simulink model "TransmissionController"  (R2026b)
StartFcn:
  | %tic
StopFcn:
  | %toc
libraries: autolibtranscontrolscommon x1
settings Model: Creator=The MathWorks, Inc.  LastModifiedBy=The MathWorks, Inc.

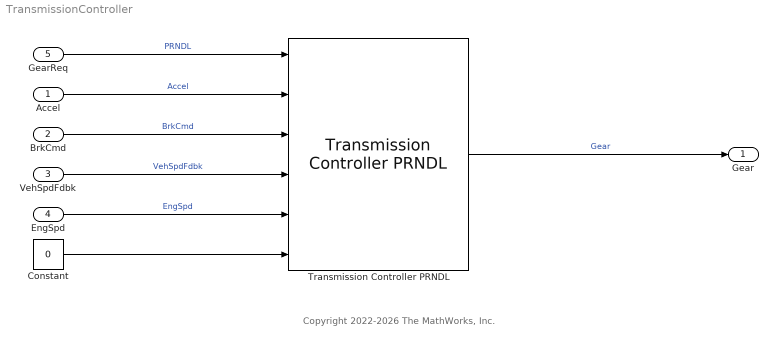
== system TransmissionController ==
  note: Copyright 2022-2026 The MathWorks, Inc.
  Accel : Inport  OutDataTypeStr=double  PortDimensions=1
  BrkCmd : Inport  Port=2  OutDataTypeStr=double  PortDimensions=1
  VehSpdFdbk : Inport  Port=3  OutDataTypeStr=double  Unit=m/s  PortDimensions=1
  EngSpd : Inport  Port=4  OutDataTypeStr=double  Unit=rad/s  PortDimensions=1
  GearReq : Inport  Port=5  OutDataTypeStr=double  PortDimensions=1
  Constant : Constant  Value=0  SampleTime=-1
  Transmission Controller PRNDL : autolibtranscontrolscommon/Transmission Controller PRNDL  DriveMode=off  GearInit=CtrlTcuInitGear  LugSpd=CtrlTcuLugSpd  MinUpSpd=CtrlTcuMinUpSpd  tClutchUp=CtrlTcuTmUpSh  tClutchDn=CtrlTcuTmDnSh  tPark=120  VelUnit=km/hr  UpShSpd=CtrlTcuUpShSpd  UpLdBpt=CtrlTcuUpLdBpt  UpShBpt=1:7  UpPtBpt=CtrlTcuUpPtBpt  DnShfSpd=CtrlTcuDnShSpd  DnShSpd=CtrlTcuDnShSpd  DnLdBpt=CtrlTcuDnLdBpt  DnShBpt=2:8  DnPtBpt=CtrlTcuDnPtBpt  POFS=CtrlTcuPedalOffset  GOFS=CtrlTcuGearOffset  Ngears=8  aMode=6
  Gear : Outport  OutDataTypeStr=double  PortDimensions=1  VectorParamsAs1DForOutWhenUnconnected=off
  wires:
  Constant/1 -> Transmission Controller PRNDL/6
  GearReq/1 -> Transmission Controller PRNDL/1  "PRNDL"
  Accel/1 -> Transmission Controller PRNDL/2  "Accel"
  BrkCmd/1 -> Transmission Controller PRNDL/3  "BrkCmd"
  EngSpd/1 -> Transmission Controller PRNDL/5  "EngSpd"
  VehSpdFdbk/1 -> Transmission Controller PRNDL/4  "VehSpdFdbk"
  Transmission Controller PRNDL/1 -> Gear/1  "Gear"
